simulink model "Aula03_ex01"  (Simulink 8.3)
settings: Solver=VariableStepDiscrete  StartTime=0.0  StopTime=0.1  RelTol=1e-3
libraries: simulink x2, dspsigops x1
settings Model: Creator=Andréa  LastModifiedBy=unieerisantos
settings OptimizationCC: ExpressionDepthLimit=2147483647
settings DebuggingCC: SolverPrmCheckMsg=none  FcnCallInpInsideContextMsg=UseLocalSettings

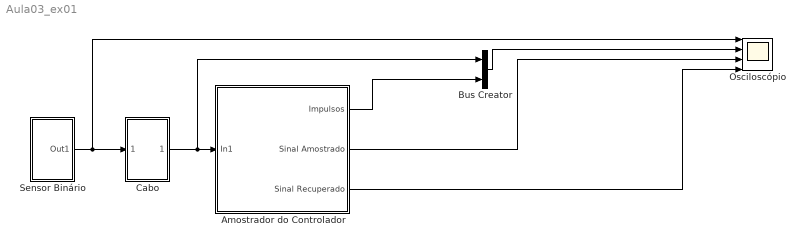
== system Aula03_ex01 ==
  Amostrador do Controlador : Subsystem
  Bus Creator : BusCreator  Inputs=2
  Cabo : Subsystem
  Osciloscópio : Scope  NumInputPorts=4
      settings: YMin=-0.5~-0.5~-1.5~-0.5  YMax=1.5~1.5~1.5~1.5
  Sensor Binário : Subsystem
  wires:
  Sensor Binário/1(Out1) -> Osciloscópio/1, Cabo/1(In1)
  Cabo/1(Out1) -> Bus Creator/1, Amostrador do Controlador/1(In1)
  Bus Creator/1 -> Osciloscópio/2
  Amostrador do Controlador/1(Impulsos) -> Bus Creator/2
  Amostrador do Controlador/2(Sinal Amostrado) -> Osciloscópio/3
  Amostrador do Controlador/3(Sinal Recuperado) -> Osciloscópio/4

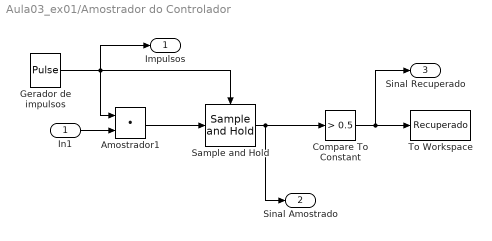
== system Aula03_ex01/Amostrador do Controlador ==
  In1 : Inport
  Amostrador1 : DotProduct  InputSameDT=on  OutDataTypeStr=Inherit: Inherit via internal rule
  Compare To Constant : simulink/Logic and Bit Operations/Compare To Constant  relop=>  const=0.5  OutDataTypeStr=uint8
  Gerador de impulsos : DiscretePulseGenerator  PulseType=Time based  Period=0.001  PhaseDelay=0.0005
  Sample and Hold : dspsigops/Sample and Hold  trig=Rising edge  initCond=0  latchinput=off
  To Workspace : ToWorkspace  VariableName=Recuperado  SampleTime=0.001
  Impulsos : Outport
  Sinal Amostrado : Outport  Port=2
  Sinal Recuperado : Outport  Port=3
  wires:
  Sample and Hold/1 -> Compare To Constant/1, Sinal Amostrado/1
  Compare To Constant/1 -> To Workspace/1, Sinal Recuperado/1
  Amostrador1/1 -> Sample and Hold/1
  Gerador de impulsos/1 -> Sample and Hold/Trigger, Amostrador1/1, Impulsos/1
  In1/1 -> Amostrador1/2

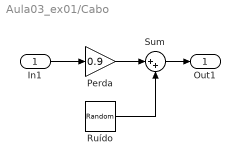
== system Aula03_ex01/Cabo ==
  In1 : Inport
  Perda : Gain  Gain=0.9
  Ruído : RandomNumber  Variance=0.7  Seed=150  SampleTime=1e-4
  Sum : Sum  Inputs=|++
  Out1 : Outport
  wires:
  Perda/1 -> Sum/1
  Ruído/1 -> Sum/2
  In1/1 -> Perda/1
  Sum/1 -> Out1/1

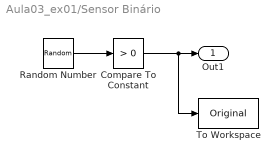
== system Aula03_ex01/Sensor Binário ==
  Compare To Constant : simulink/Logic and Bit Operations/Compare To Constant  relop=>  const=0  OutDataTypeStr=uint8
  Random Number : RandomNumber  Seed=10  SampleTime=0.001
  To Workspace : ToWorkspace  VariableName=Original  SampleTime=0.001
  Out1 : Outport
  wires:
  Random Number/1 -> Compare To Constant/1
  Compare To Constant/1 -> Out1/1, To Workspace/1
